simulink model "FocESMOGenerator"  (R2024a)
settings: Solver=FixedStepDiscrete  StartTime=0.0  StopTime=5  FixedStep=0.00005  RelTol=1e-3
values from neighbouring files (symbols this model uses):
  Ld = 5.135e-05    [ASMO_HFI_Generator.mat]
  Max_Current = 10    [ASMO_HFI_Generator.mat]
  Pole = 10    [ASMO_HFI_Generator.mat]
  Rs = 0.082    [ASMO_HFI_Generator.mat]
  Switch_Speed = 500    [ASMO_HFI_Generator.mat]
  UdInjectVal = 2.5    [ASMO_HFI_Generator.mat]
undefined symbols (not defined in the file or in its folder): DiscIntNeverNeededParam
libraries: slpidlib x5
(part 1 of 2)
settings Model: Creator=张先生  LastModifiedBy=张先生
settings OptimizationCC: DefaultParameterBehavior=Inlined  UseDivisionForNetSlopeComputation=on  GainParamInheritBuiltInType=on  UseFloatMulNetSlope=on  InlineInvariantSignals=on  PassReuseOutputArgsAs=Individual arguments  ZeroExternalMemoryAtStartup=off  ZeroInternalMemoryAtStartup=off  NoFixptDivByZeroProtection=on  EfficientFloat2IntCast=on  LifeSpan=1  OptimizeBlockOrder=speed  DifferentSizesBufferReuse=on  EfficientTunableParamExpr=on
settings DebuggingCC: ParameterTunabilityLossMsg=error
settings HardwareCC: ProdBitPerPointer=32  ProdBitPerSizeT=32  ProdBitPerPtrDiffT=32  ProdLargestAtomicInteger=Long  ProdLargestAtomicFloat=Double  ProdWordSize=32  ProdLongLongMode=on  ProdHWDeviceType=ARM Compatible->ARM Cortex-M
settings SFSimCC: MATLABDynamicMemAlloc=off
settings RTWCC: Description=Embedded Coder  SystemTargetFile=ert.tlc  GenCodeOnly=on  TemplateMakefile=ert_default_tmf  GenerateReport=on  LaunchReport=on
settings CodeAppCC: ForceParamTrailComments=on  IgnoreCustomStorageClasses=off  OperatorAnnotations=on  SimulinkDataObjDesc=on  SFDataObjDesc=on  CustomSymbolStrGlobalVar=rt$N$M  CustomSymbolStrType=$N$M  CustomSymbolStrFcn=$N$M$F  CustomSymbolStrMacro=$N$M  InsertBlockDesc=on
settings ERTTargetCC: TargetLangStandard=C99 (ISO)  CodeReplacementLibrary=ARM Cortex-M  GenerateSampleERTMain=on  IncludeMdlTerminateFcn=off  CombineSignalStateStructs=on  SupportComplex=off  SupportContinuousTime=on  InlinedParameterPlacement=NonHierarchical  ERTCustomFileTemplate=example_file_process.tlc  ERTFilePackagingFormat=CompactWithDataFile

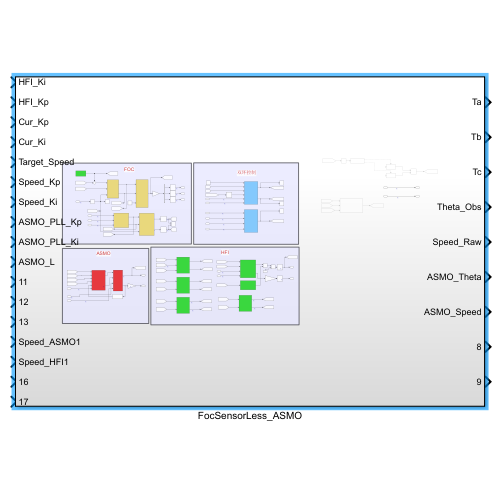
[thumbnail: Simulink's stored preview of the top-level diagram]
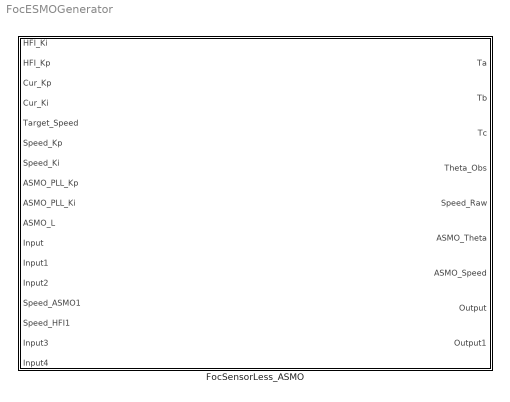
== system FocESMOGenerator ==
  FocSensorLess_ASMO : Subsystem

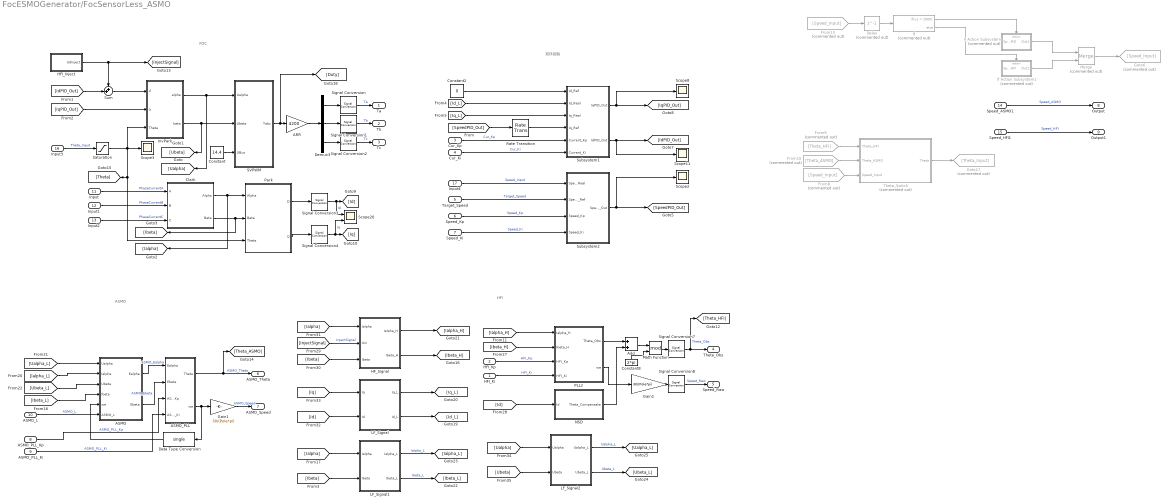
== system FocESMOGenerator/FocSensorLess_ASMO ==
  note: ASMO
  note: HFI
  note: 双环控制
  note: FOC
  HFI_Ki : Inport
  HFI_Kp : Inport  Port=2
  Cur_Kp : Inport  Port=3
  Cur_Ki : Inport  Port=4
  Target_Speed : Inport  Port=5
  Speed_Kp : Inport  Port=6
  Speed_Ki : Inport  Port=7
  ASMO_PLL_Kp : Inport  Port=8
  ASMO_PLL_Ki : Inport  Port=9
  ASMO_L : Inport  Port=10
  Input : Inport  Port=11
  Input1 : Inport  Port=12
  Input2 : Inport  Port=13
  Speed_ASMO1 : Inport  Port=14
  Speed_HFI1 : Inport  Port=15
  Input3 : Inport  Port=16
  Input4 : Inport  Port=17
  ARR : Gain  Gain=4200
  ASMO : Subsystem
  ASMO_PLL : Subsystem
  Add : Sum  OutDataTypeStr=single  AccumDataTypeStr=single
  Clark : Subsystem  TreatAsAtomicUnit=on
      settings: RTWSystemCode=Inline  RTWFcnNameOpts=Use subsystem name
      mask Display:
      | port_label('input',1,'a','texmode','on');
      | port_label('input',2,'b','texmode','on');
      | port_label('input',3,'c','texmode','on');
      | 
      | port_label('output',1,'\alpha','texmode','on');
      | port_label('output',2,'\beta','texmode','on');
      | 
      | fprintf('Clark');
  Constant : Constant  Value=14.4  OutDataTypeStr=single
  Constant2 : Constant  Value=0  OutDataTypeStr=single
  Constant8 : Constant  Value=2*pi  OutDataTypeStr=single
  Data Type Conversion : DataTypeConversion  OutDataTypeStr=single  SaturateOnIntegerOverflow=off  RndMeth=Floor
  Delay : Delay  Commented=on  DelayLength=1
  Demux3 : Demux  Outputs=3
  From10 : From  Commented=on  GotoTag=Theta_ASMO
  From13 : From  Commented=on  GotoTag=Speed_Input
  From8 : From  Commented=on  GotoTag=Speed_Input
  From9 : From  Commented=on  GotoTag=Theta_HFI
  Gain1 : Gain  Gain=30/(Pole*pi)
  Gain2 : Gain  Gain=30/(Pole*pi)  OutDataTypeStr=single
  Goto17 : Goto  Commented=on  GotoTag=Theta_Input
  Goto6 : Goto  Commented=on  GotoTag=Speed_Input
  HFI_Inject : Subsystem
  HF_Signal : Subsystem
  If : If  Commented=on  IfExpression=u1 > 1000
  If Action Subsystem : Subsystem  Commented=on  TreatAsAtomicUnit=on
  If Action Subsystem1 : Subsystem  Commented=on  TreatAsAtomicUnit=on
  InvPark : Subsystem  TreatAsAtomicUnit=on
      settings: RTWFcnNameOpts=Use subsystem name
      mask Display:
      | port_label('input',1,'d','texmode','on');
      | port_label('input',2,'q','texmode','on');
      | port_label('input',3,'\theta','texmode','on');
      | 
      | port_label('output',1,'\alpha','texmode','on');
      | port_label('output',2,'\beta','texmode','on');
      | 
      | fprintf('Inverse\nPark')
  LF_Signal : Subsystem
  LF_Signal1 : Subsystem
  LF_Signal2 : Subsystem
  Math Function : Math  Operator=mod
  Merge : Merge  Commented=on
  NSD : Subsystem
  PLL2 : Subsystem
  Park : Subsystem  TreatAsAtomicUnit=on
      settings: RTWFcnNameOpts=Use subsystem name
      mask Display:
      | port_label('input',1,'\alpha','texmode','on');
      | port_label('input',2, '\beta','texmode','on');
      | port_label('input',3, '\theta','texmode','on');
      | 
      | port_label('output',1,'d','texmode','on');
      | port_label('output',2,'q','texmode','on');
      | fprintf('Park');
  Rate Transition : RateTransition
  SVPWM : Subsystem  TreatAsAtomicUnit=on
  Saturation : Saturate  UpperLimit=2*pi-0.001  LowerLimit=-2*pi + 0.001
  Scope{2..3,8,11} (4 alike) : Scope
  Scope20 : Scope  NumInputPorts=2
  Signal Conversion{,1..4,7..8} (7 alike) : SignalConversion  OverrideOpt=off
  Subsystem1 : Subsystem
  Subsystem2 : Subsystem
  Sum : Sum  Inputs=++|
  Theta_Switch : Subsystem  Commented=on
  Ta : Outport
  Tb : Outport  Port=2
  Tc : Outport  Port=3
  Theta_Obs : Outport  Port=4
  Speed_Raw : Outport  Port=5
  ASMO_Theta : Outport  Port=6
  ASMO_Speed : Outport  Port=7
  Output : Outport  Port=8
  Output1 : Outport  Port=9
  wires:
  InvPark/1(alpha) -> SVPWM/1(Ualpha), [Ualpha]
  InvPark/2(beta) -> SVPWM/2(Ubeta), [Ubeta]
  Saturation/1 -> [Theta], Park/3(Theta), Scope3/1, InvPark/3(Theta)
  SVPWM/1(Tabc) -> [Duty], ARR/1
  ARR/1 -> Demux3/1
  Park/1(D) -> Signal Conversion3/1
  Signal Conversion4/1 -> Scope20/2, [Iq]  "Iq"
  Signal Conversion2/1 -> Tc/1  "Tc"
  Signal Conversion3/1 -> Scope20/1, [Id]  "Id"
  Signal Conversion/1 -> Ta/1  "Ta"
  Demux3/2 -> Signal Conversion1/1
  Demux3/1 -> Signal Conversion/1
  Park/2(Q) -> Signal Conversion4/1
  Demux3/3 -> Signal Conversion2/1
  Signal Conversion1/1 -> Tb/1  "Tb"
  Constant/1 -> SVPWM/3(UBus)
  Clark/2(Beta) -> [Ibeta], Park/2(Beta)
  Clark/1(Alpha) -> [Ialpha], Park/1(Alpha)
  [IqPID_Out] -> InvPark/2(q)
  Input3/1 -> Saturation/1  "Theta_Input"
  Gain1/1 -> ASMO_Speed/1  "ASMO_Speed"
  [Ialpha_L] -> ASMO/2(Ialpha)
  ASMO/2(Ebeta) -> ASMO_PLL/2(Ebeta)  "ASMO_Ebeta"
  ASMO_PLL/2(we) -> Gain1/1, Data Type Conversion/1
  ASMO/1(Ealpha) -> ASMO_PLL/1(Ealpha)  "ASMO_Ealpha"
  ASMO_PLL/1(Theta) -> [Theta_ASMO], ASMO_Theta/1  "ASMO_Theta"
  [Ualpha_L] -> ASMO/1(Ualpha)
  [Ubeta_L] -> ASMO/3(Ubeta)
  [Ibeta_L] -> ASMO/4(Ibeta)
  Data Type Conversion/1 -> ASMO/5(we)
  HFI_Inject/1(UdInject) -> Sum/1, [InjectSignal]
  [IdPID_Out] -> Sum/2
  Sum/1 -> InvPark/1(d)
  Gain2/1 -> Signal Conversion8/1
  [Ibeta_H] -> PLL2/2(Ibeta_H)
  PLL2/2(we) -> Gain2/1
  LF_Signal/2(Id_L) -> [Id_L]
  Add/1 -> Math Function/1
  [Id] -> NSD/1(Id)
  [Ialpha] -> HF_Signal/1(Ialpha)
  Signal Conversion8/1 -> Speed_Raw/1  "Speed_Raw"
  LF_Signal/1(Iq_L) -> [Iq_L]
  NSD/1(Theta_Compensate) -> Add/2
  HF_Signal/2(Ibeta_H) -> [Ibeta_H]
  [Ibeta] -> HF_Signal/3(Ibeta)
  [Id] -> LF_Signal/2(Id)
  HF_Signal/1(Ialpha_H) -> [Ialpha_H]
  [Iq] -> LF_Signal/1(Iq)
  HFI_Kp/1 -> PLL2/3(HFI_Kp)  "HFI_Kp"
  PLL2/1(Theta_Obs) -> Add/1
  Constant8/1 -> Math Function/2
  [Ialpha_H] -> PLL2/1(Ialpha_H)
  [InjectSignal] -> HF_Signal/2(Uin)  "InjectSignal"
  HFI_Ki/1 -> PLL2/4(HFI_Ki)  "HFI_Ki"
  Math Function/1 -> Signal Conversion7/1
  Signal Conversion7/1 -> [Theta_HFI], Theta_Obs/1  "Theta_Obs"
  [Iq_L] -> Subsystem1/3(Iq_Real)
  Cur_Kp/1 -> Subsystem1/5(Current_Kp)  "Cur_Kp"
  Speed_Kp/1 -> Subsystem2/3(Speed_Kp)  "Speed_Kp"
  Constant2/1 -> Subsystem1/1(Id_Ref)
  Subsystem2/1(SpeedPID_Out) -> Scope2/1, [SpeedPID_Out]
  Speed_Ki/1 -> Subsystem2/4(Speed_Ki)  "Speed_Ki"
  Input4/1 -> Subsystem2/1(Speed_Real)  "Speed_Input"
  [SpeedPID_Out] -> Rate Transition/1
  Cur_Ki/1 -> Subsystem1/6(Current_Ki)  "Cur_Ki"
  Rate Transition/1 -> Subsystem1/4(Iq_Ref)
  Target_Speed/1 -> Subsystem2/2(Speed_Ref)  "Target_Speed"
  Subsystem1/2(IdPID_Out) -> Scope11/1, [IdPID_Out]
  Subsystem1/1(IqPID_Out) -> Scope8/1, [IqPID_Out]
  [Id_L] -> Subsystem1/2(Id_Real)
  ASMO_PLL_Kp/1 -> ASMO_PLL/3(ASMO_PLL_Kp)  "ASMO_PLL_Kp"
  ASMO_PLL_Ki/1 -> ASMO_PLL/4(ASMO_PLL_Ki)  "ASMO_PLL_Ki"
  ASMO_L/1 -> ASMO/6(ASMO_L)  "ASMO_L"
  [Ibeta] -> LF_Signal1/2(Ibeta)
  [Ialpha] -> LF_Signal1/1(Ialpha)
  LF_Signal1/1(Ialpha_L) -> [Ialpha_L]  "Ialpha_L"
  LF_Signal1/2(Ibeta_L) -> [Ibeta_L]  "Ibeta_L"
  [Ubeta] -> LF_Signal2/2(Ubeta)
  LF_Signal2/2(Ubeta_L) -> [Ubeta_L]  "Ubeta_L"
  LF_Signal2/1(Ualpha_L) -> [Ualpha_L]  "Ualpha_L"
  [Ualpha] -> LF_Signal2/1(Ualpha)
  Input/1 -> Clark/1(A)  "PhaseCurrentA"
  Input2/1 -> Clark/3(C)  "PhaseCurrentC"
  Input1/1 -> Clark/2(B)  "PhaseCurrentB"
  From8/1 -> Theta_Switch/3(Speed_Input)
  From10/1 -> Theta_Switch/2(Theta_ASMO)
  From9/1 -> Theta_Switch/1(Theta_HFI)
  Theta_Switch/1(Theta) -> Goto17/1
  If/1 -> If Action Subsystem/Action
  If/2 -> If Action Subsystem1/Action
  If Action Subsystem/1(Out1) -> Merge/1
  If Action Subsystem1/1(Out1) -> Merge/2
  Merge/1 -> Goto6/1
  From13/1 -> Delay/1
  Delay/1 -> If/1
  Speed_HFI1/1 -> Output1/1  "Speed_HFI"
  Speed_ASMO1/1 -> Output/1  "Speed_ASMO"

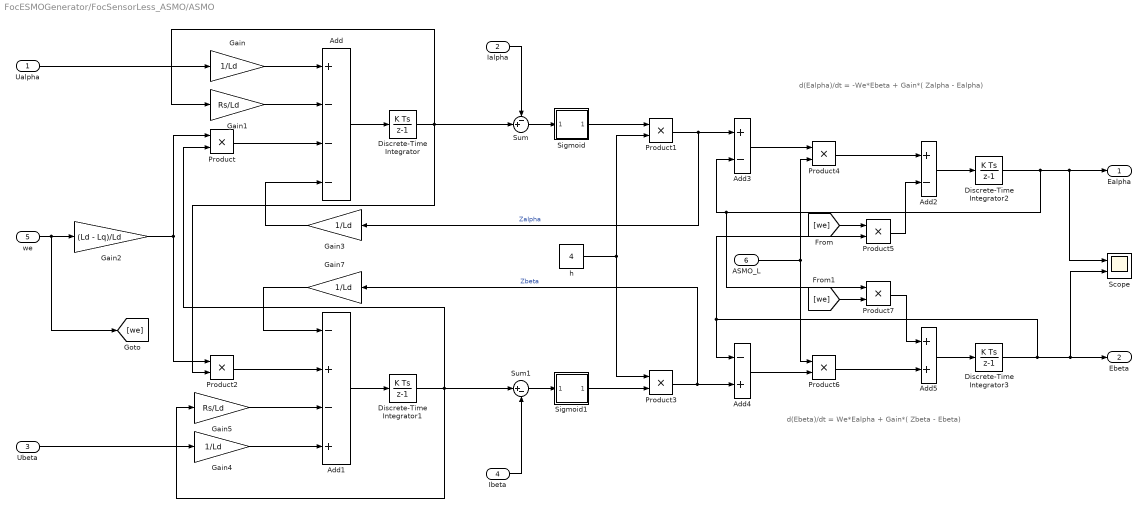
== system FocESMOGenerator/FocSensorLess_ASMO/ASMO ==
  note: d(Ealpha)/dt = -We*Ebeta + Gain*( Zalpha - Ealpha)
  note: d(Ebeta)/dt = We*Ealpha + Gain*( Zbeta - Ebeta)
  Ualpha : Inport
  Ialpha : Inport  Port=2
  Ubeta : Inport  Port=3
  Ibeta : Inport  Port=4
  we : Inport  Port=5
  ASMO_L : Inport  Port=6
  Add : Sum  Inputs=+---  OutDataTypeStr=single  AccumDataTypeStr=single
  Add1 : Sum  Inputs=-+-+  OutDataTypeStr=single  AccumDataTypeStr=single
  Add2 : Sum  Inputs=+-  OutDataTypeStr=single  AccumDataTypeStr=single
  Add3 : Sum  Inputs=+-  OutDataTypeStr=single  AccumDataTypeStr=single
  Add4 : Sum  Inputs=-+  OutDataTypeStr=single  AccumDataTypeStr=single
  Add5 : Sum  OutDataTypeStr=single  AccumDataTypeStr=single
  Discrete-Time Integrator{,1..3} (4 alike) : DiscreteIntegrator  SampleTime=-1  OutDataTypeStr=single  ICPrevOutput=DiscIntNeverNeededParam  ICPrevScaledInput=DiscIntNeverNeededParam
  Gain{,3..4,7} (4 alike) : Gain  Gain=1/Ld  OutDataTypeStr=single
  Gain1 : Gain  Gain=Rs/Ld  OutDataTypeStr=single
  Gain2 : Gain  Gain=(Ld - Lq)/Ld
  Gain5 : Gain  Gain=Rs/Ld  OutDataTypeStr=single
  Product{,1..6} (7 alike) : Product  OutDataTypeStr=single
  Product7 : Product
  Scope : Scope  NumInputPorts=2
  Sigmoid : Subsystem
  Sigmoid1 : Subsystem
  Sum : Sum  Inputs=-+|
  Sum1 : Sum  Inputs=|+-
  h : Constant  Value=4  OutDataTypeStr=single
  Ealpha : Outport
  Ebeta : Outport  Port=2
  wires:
  Gain/1 -> Add/1
  Gain1/1 -> Add/2
  Ualpha/1 -> Gain/1
  Add/1 -> Discrete-Time Integrator/1
  Product/1 -> Add/3
  Gain2/1 -> Product2/1, Product/1
  Discrete-Time Integrator/1 -> Product2/2, Sum/2, Gain1/1
  Ialpha/1 -> Sum/1
  Sum/1 -> Sigmoid/1(In1)
  Sigmoid/1(Out1) -> Product1/1
  h/1 -> Product3/1, Product1/2
  Product1/1 -> Add3/1, Gain3/1  "Zalpha"
  Gain3/1 -> Add/4
  Add1/1 -> Discrete-Time Integrator1/1
  Product3/1 -> Add4/2, Gain7/1  "Zbeta"
  Sum1/1 -> Sigmoid1/1(In1)
  Discrete-Time Integrator1/1 -> Sum1/1, Gain5/1, Product/2
  Ibeta/1 -> Sum1/2
  Sigmoid1/1(Out1) -> Product3/2
  Gain4/1 -> Add1/4
  Gain5/1 -> Add1/3
  Product2/1 -> Add1/2
  Gain7/1 -> Add1/1
  Ubeta/1 -> Gain4/1
  Add3/1 -> Product4/1
  Product4/1 -> Add2/1
  Add2/1 -> Discrete-Time Integrator2/1
  Discrete-Time Integrator2/1 -> Ealpha/1, Scope/1, Product7/1, Add3/2
  ASMO_L/1 -> Product4/2, Product6/1
  Product5/1 -> Add2/2
  [we] -> Product5/1
  Add4/1 -> Product6/2
  Product6/1 -> Add5/2
  [we] -> Product7/2
  Product7/1 -> Add5/1
  Add5/1 -> Discrete-Time Integrator3/1
  Discrete-Time Integrator3/1 -> Product5/2, Add4/1, Scope/2, Ebeta/1
  we/1 -> [we], Gain2/1

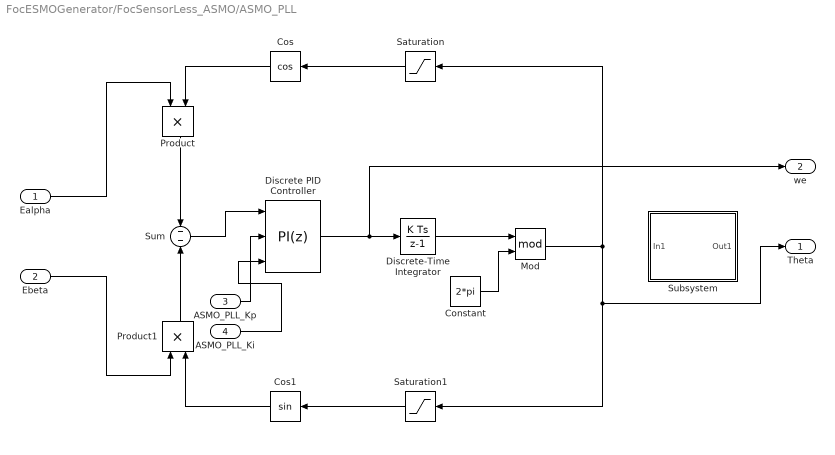
== system FocESMOGenerator/FocSensorLess_ASMO/ASMO_PLL ==
  Ealpha : Inport
  Ebeta : Inport  Port=2
  ASMO_PLL_Kp : Inport  Port=3
  ASMO_PLL_Ki : Inport  Port=4
  Constant : Constant  Value=2*pi  OutDataTypeStr=single
  Cos : Trigonometry  Operator=cos  ApproximationMethod=Lookup
  Cos1 : Trigonometry  ApproximationMethod=Lookup
  Discrete PID Controller : slpidlib/PID Controller  Controller=PI  Form=Parallel  TimeDomain=Discrete-time  UseExternalTs=off  SampleTime=-1  IntegratorMethod=Forward Euler  FilterMethod=Forward Euler  ControllerParametersSource=external  P=10  I=1000  UseKiTs=off  D=0  UseExternalDerivativeSource=off  N=100  UseFilter=on  TunerSelectOption=Transfer Function Based (PID Tuner App)  InitialConditionSource=internal  InitialConditionForIntegrator=0  InitialConditionForFilter=0  DifferentiatorICPrevScaledInput=0  ExternalReset=none  TrackingMode=off  Kt=1  LimitOutput=off  SatLimitsSource=internal  UpperSaturationLimit=pi*2  LowerSaturationLimit=-pi*2  LinearizeAsGain=on  AntiWindupMode=clamping  Kb=1  LimitIntegrator=off  UpperIntegratorSaturationLimit=inf  LowerIntegratorSaturationLimit=-inf  PGainOutDataTypeStr=single  PProdOutDataTypeStr=single  POutMin=[]  POutMax=[]  IGainOutDataTypeStr=single  IProdOutDataTypeStr=single  IOutMin=[]  IOutMax=[]  DOutMin=[]  DOutMax=[]  NOutMin=[]  NOutMax=[]  SumOutDataTypeStr=single  SumOutMin=[]  SumOutMax=[]  SaturationOutMin=[]  SaturationOutMax=[]  PParamMin=[]  PParamMax=[]  IParamMin=[]  IParamMax=[]  DParamMin=[]  DParamMax=[]  NParamMin=[]  NParamMax=[]  KbParamMin=[]  KbParamMax=[]  KtParamMin=[]  KtParamMax=[]  KbOutMin=[]  KbOutMax=[]  KtOutMin=[]  KtOutMax=[]  IntegratorOutMin=[]  IntegratorOutMax=[]  FilterOutMin=[]  FilterOutMax=[]  SumI1OutMin=[]  SumI1OutMax=[]  SumI2OutMin=[]  SumI2OutMax=[]  SumI3OutMin=[]  SumI3OutMax=[]  SumI4OutMin=[]  SumI4OutMax=[]  SumDOutMin=[]  SumDOutMax=[]  DifferentiatorOutMin=[]  DifferentiatorOutMax=[]  FilterDiffOutCoefMin=[]  FilterDiffOutCoefMax=[]  ReciprocalOutMin=[]  ReciprocalOutMax=[]  SumDenOutMin=[]  SumDenOutMax=[]  SumNumOutMin=[]  SumNumOutMax=[]  DivideOutMin=[]  DivideOutMax=[]  UdiffTsProdOutMin=[]  UdiffTsProdOutMax=[]  NTsProdOutMin=[]  NTsProdOutMax=[]  UintegralTsProdOutMin=[]  UintegralTsProdOutMax=[]  UngainTsProdOutMin=[]  UngainTsProdOutMax=[]  ClampingZeroOutDataTypeStr=Inherit: Inherit via back propagation  ClampingZeroOutMin=[]  ClampingZeroOutMax=[]  FilterDenConstantOutDataTypeStr=Inherit: Inherit via back propagation  FilterDenConstantOutMin=[]  FilterDenConstantOutMax=[]  PCopyOutDataTypeStr=Inherit: Inherit via back propagation  PCopyOutMin=[]  PCopyOutMax=[]  NCopyOutDataTypeStr=Inherit: Inherit via back propagation  NCopyOutMin=[]  NCopyOutMax=[]  IntegratorContinuousStateAttributes=''  IntegratorStateMustResolveToSignalObject=off  IntegratorRTWStateStorageClass=Auto  FilterContinuousStateAttributes=''  FilterStateMustResolveToSignalObject=off  FilterRTWStateStorageClass=Auto  ParallelPVariant=ExternalParameters  IdealPVariant=Disabled  IVariant=ExternalParameters  DVariant=Disabled  IntegratorVariant=Discrete  SatVariant=Disabled  AWVariant=Passthrough  PCopyVariant=Disabled  TRVariant=Disabled  FdbkBlocksVariant=Forward  IdealPFdbkVariant=Disabled  SatFdbkVariant=Disabled  DerivativeFilterVariant=Disabled  NVariant=Disabled  NCopyVariant=Disabled_SignalSpec  FilterICVariant=Disabled  IntegratorICVariant=InternalICs  ExternalResetVariant=Disabled  TRSumVariant=Passthrough  SumFdbkVariant=Disabled  SumVariant=Sum_PI  TsampFilterVariant=InternalTs  TsampNgainVariant=Passthrough  TsampIntegralVariant=Disabled_SignalSpec  ExternalSaturationOutDataTypeStr=Inherit: Same as second input  DerivativeSourceVariant=Disabled
      settings: LibrarySourceBlock=simulink/Discrete/Discrete PID Controller
  Discrete-Time Integrator : DiscreteIntegrator  SampleTime=-1  OutDataTypeStr=single  ICPrevOutput=DiscIntNeverNeededParam  ICPrevScaledInput=DiscIntNeverNeededParam
  Mod : Math  Operator=mod
  Product : Product  OutDataTypeStr=single
  Product1 : Product  OutDataTypeStr=single
  Saturation : Saturate  UpperLimit=2*pi - 0.001  LowerLimit=-2*pi + 0.001
  Saturation1 : Saturate  UpperLimit=2*pi - 0.001  LowerLimit=-2*pi + 0.001
  Subsystem : Subsystem
  Sum : Sum  Inputs=-|-
  Theta : Outport
  we : Outport  Port=2
  wires:
  Ebeta/1 -> Product1/1
  Ealpha/1 -> Product/1
  Product/1 -> Sum/1
  Product1/1 -> Sum/2
  Sum/1 -> Discrete PID Controller/1
  Discrete-Time Integrator/1 -> Mod/1
  Constant/1 -> Mod/2
  Mod/1 -> Theta/1, Saturation1/1, Saturation/1
  Saturation/1 -> Cos/1
  Cos/1 -> Product/2
  Saturation1/1 -> Cos1/1
  Cos1/1 -> Product1/2
  Discrete PID Controller/1 -> we/1, Discrete-Time Integrator/1
  ASMO_PLL_Kp/1 -> Discrete PID Controller/2
  ASMO_PLL_Ki/1 -> Discrete PID Controller/3

== system FocESMOGenerator/FocSensorLess_ASMO/Clark ==
  A : Inport  OutDataTypeStr=single
  B : Inport  Port=2  OutDataTypeStr=single
  C : Inport  Port=3  OutDataTypeStr=single
  Gain : Gain  Gain=single(2/3)  OutDataTypeStr=single
  Gain1 : Gain  Gain=0.5  OutDataTypeStr=single
  Gain2 : Gain  Gain=single(sqrt(3)/3)  OutDataTypeStr=single
  Sum : Sum  Inputs=|++  OutDataTypeStr=single
  Sum1 : Sum  Inputs=|+-  OutDataTypeStr=single
  Sum2 : Sum  Inputs=+-|  OutDataTypeStr=single
  Alpha : Outport  OutDataTypeStr=single
  Beta : Outport  Port=2  OutDataTypeStr=single
  wires:
  Sum/1 -> Gain1/1
  Gain2/1 -> Beta/1
  B/1 -> Sum2/1, Sum/1
  Gain1/1 -> Sum1/2
  Gain/1 -> Alpha/1
  Sum2/1 -> Gain2/1
  C/1 -> Sum2/2, Sum/2
  A/1 -> Sum1/1
  Sum1/1 -> Gain/1

== system FocESMOGenerator/FocSensorLess_ASMO/HFI_Inject ==
  note: 前0.2S进行极性辨识
  Scope : Scope
  Scope1 : Scope  NumInputPorts=2
  Subsystem : Subsystem
  Subsystem4 : Subsystem
  Sum1 : Sum  Inputs=++|
  UdInject : Outport
  wires:
  Subsystem/1(Ud_Inject) -> Scope1/2, Sum1/2
  Subsystem4/1(NDS_Signal) -> Scope1/1, Sum1/1
  Sum1/1 -> Scope/1, UdInject/1

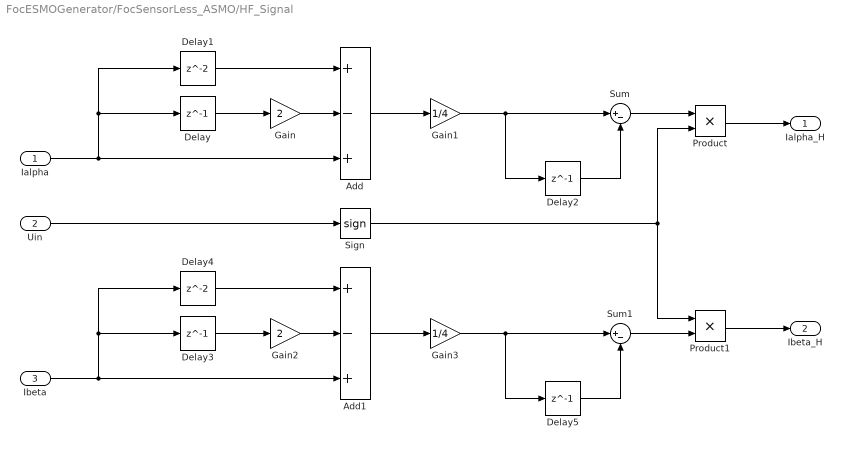
== system FocESMOGenerator/FocSensorLess_ASMO/HF_Signal ==
  Ialpha : Inport
  Uin : Inport  Port=2
  Ibeta : Inport  Port=3
  Add : Sum  Inputs=+-+  OutDataTypeStr=single  AccumDataTypeStr=single
  Add1 : Sum  Inputs=+-+  OutDataTypeStr=single  AccumDataTypeStr=single
  Delay{,2..3,5} (4 alike) : Delay  DelayLength=1
  Delay1 : Delay
  Delay4 : Delay
  Gain : Gain  Gain=2  OutDataTypeStr=single
  Gain1 : Gain  Gain=1/4  OutDataTypeStr=single
  Gain2 : Gain  Gain=2  OutDataTypeStr=single
  Gain3 : Gain  Gain=1/4  OutDataTypeStr=single
  Product : Product  OutDataTypeStr=single
  Product1 : Product  OutDataTypeStr=single
  Sign : Signum
  Sum : Sum  Inputs=|+-
  Sum1 : Sum  Inputs=|+-
  Ialpha_H : Outport
  Ibeta_H : Outport  Port=2
  wires:
  Delay/1 -> Gain/1
  Delay1/1 -> Add/1
  Gain/1 -> Add/2
  Ialpha/1 -> Add/3, Delay1/1, Delay/1
  Add/1 -> Gain1/1
  Gain1/1 -> Delay2/1, Sum/1
  Delay2/1 -> Sum/2
  Sum/1 -> Product/1
  Product/1 -> Ialpha_H/1
  Uin/1 -> Sign/1
  Sign/1 -> Product1/1, Product/2
  Product1/1 -> Ibeta_H/1
  Add1/1 -> Gain3/1
  Delay5/1 -> Sum1/2
  Gain3/1 -> Delay5/1, Sum1/1
  Delay4/1 -> Add1/1
  Gain2/1 -> Add1/2
  Ibeta/1 -> Add1/3, Delay4/1, Delay3/1
  Delay3/1 -> Gain2/1
  Sum1/1 -> Product1/2

== system FocESMOGenerator/FocSensorLess_ASMO/If Action Subsystem ==
  Speed_ASMO : Inport
  Action Port : ActionPort  ActionPortLabel=if(u1 > 1000)
  Out1 : Outport
  wires:
  Speed_ASMO/1 -> Out1/1

== system FocESMOGenerator/FocSensorLess_ASMO/If Action Subsystem1 ==
  Speed_HFI : Inport
  Action Port : ActionPort  ActionPortLabel=else
  Out1 : Outport
  wires:
  Speed_HFI/1 -> Out1/1

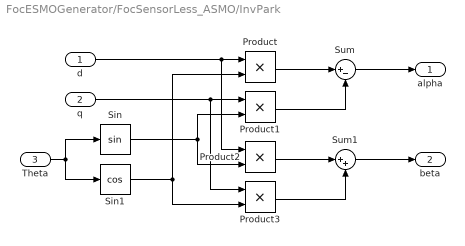
== system FocESMOGenerator/FocSensorLess_ASMO/InvPark ==
  d : Inport  OutDataTypeStr=single
  q : Inport  Port=2  OutDataTypeStr=single
  Theta : Inport  Port=3  OutDataTypeStr=single
  Product{,1..3} (4 alike) : Product  OutDataTypeStr=single
  Sin : Trigonometry  ApproximationMethod=Lookup  TableDataTypeStr=single
  Sin1 : Trigonometry  Operator=cos  ApproximationMethod=Lookup  TableDataTypeStr=single
  Sum : Sum  Inputs=|+-  OutDataTypeStr=single
  Sum1 : Sum  Inputs=|++  OutDataTypeStr=single
  alpha : Outport  OutDataTypeStr=single
  beta : Outport  Port=2  OutDataTypeStr=single
  wires:
  Sum/1 -> alpha/1
  Theta/1 -> Sin1/1, Sin/1
  d/1 -> Product2/1, Product/1
  Sin1/1 -> Product/2, Product3/2
  q/1 -> Product3/1, Product1/1
  Sin/1 -> Product1/2, Product2/2
  Product/1 -> Sum/1
  Product1/1 -> Sum/2
  Product2/1 -> Sum1/1
  Product3/1 -> Sum1/2
  Sum1/1 -> beta/1

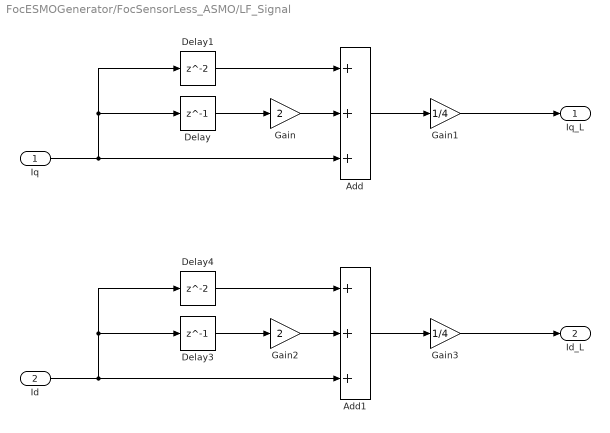
== system FocESMOGenerator/FocSensorLess_ASMO/LF_Signal ==
  Iq : Inport
  Id : Inport  Port=2
  Add : Sum  Inputs=+++  OutDataTypeStr=single  AccumDataTypeStr=single
  Add1 : Sum  Inputs=+++  OutDataTypeStr=single  AccumDataTypeStr=single
  Delay : Delay  DelayLength=1
  Delay1 : Delay
  Delay3 : Delay  DelayLength=1
  Delay4 : Delay
  Gain : Gain  Gain=2
  Gain1 : Gain  Gain=1/4  OutDataTypeStr=single
  Gain2 : Gain  Gain=2
  Gain3 : Gain  Gain=1/4  OutDataTypeStr=single
  Iq_L : Outport
  Id_L : Outport  Port=2
  wires:
  Delay/1 -> Gain/1
  Delay1/1 -> Add/1
  Gain/1 -> Add/2
  Iq/1 -> Add/3, Delay1/1, Delay/1
  Add/1 -> Gain1/1
  Gain1/1 -> Iq_L/1
  Gain3/1 -> Id_L/1
  Add1/1 -> Gain3/1
  Delay4/1 -> Add1/1
  Gain2/1 -> Add1/2
  Id/1 -> Add1/3, Delay4/1, Delay3/1
  Delay3/1 -> Gain2/1

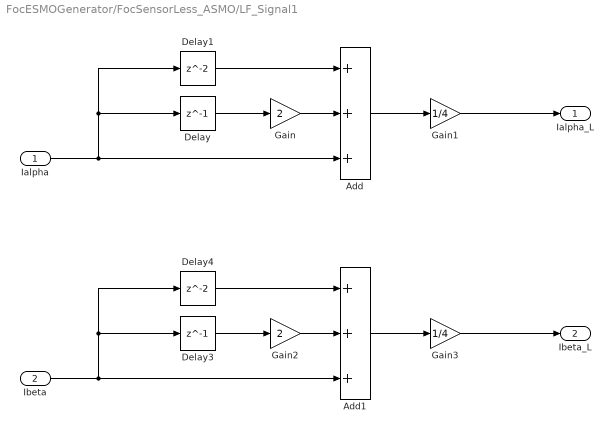
== system FocESMOGenerator/FocSensorLess_ASMO/LF_Signal1 ==
  Ialpha : Inport
  Ibeta : Inport  Port=2
  Add : Sum  Inputs=+++  OutDataTypeStr=single  AccumDataTypeStr=single
  Add1 : Sum  Inputs=+++  OutDataTypeStr=single  AccumDataTypeStr=single
  Delay : Delay  DelayLength=1
  Delay1 : Delay
  Delay3 : Delay  DelayLength=1
  Delay4 : Delay
  Gain : Gain  Gain=2  OutDataTypeStr=single
  Gain1 : Gain  Gain=1/4  OutDataTypeStr=single
  Gain2 : Gain  Gain=2  OutDataTypeStr=single
  Gain3 : Gain  Gain=1/4  OutDataTypeStr=single
  Ialpha_L : Outport
  Ibeta_L : Outport  Port=2
  wires:
  Delay/1 -> Gain/1
  Delay1/1 -> Add/1
  Gain/1 -> Add/2
  Ialpha/1 -> Add/3, Delay1/1, Delay/1
  Add/1 -> Gain1/1
  Gain1/1 -> Ialpha_L/1
  Gain3/1 -> Ibeta_L/1
  Add1/1 -> Gain3/1
  Delay4/1 -> Add1/1
  Gain2/1 -> Add1/2
  Ibeta/1 -> Add1/3, Delay4/1, Delay3/1
  Delay3/1 -> Gain2/1

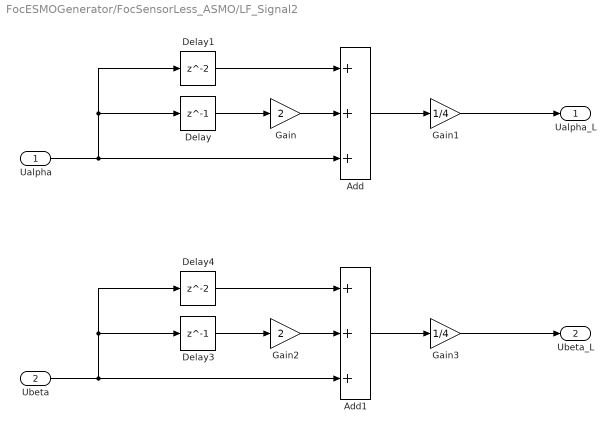
== system FocESMOGenerator/FocSensorLess_ASMO/LF_Signal2 ==
  Ualpha : Inport
  Ubeta : Inport  Port=2
  Add : Sum  Inputs=+++  OutDataTypeStr=single  AccumDataTypeStr=single
  Add1 : Sum  Inputs=+++  OutDataTypeStr=single  AccumDataTypeStr=single
  Delay : Delay  DelayLength=1
  Delay1 : Delay
  Delay3 : Delay  DelayLength=1
  Delay4 : Delay
  Gain : Gain  Gain=2  OutDataTypeStr=single
  Gain1 : Gain  Gain=1/4  OutDataTypeStr=single
  Gain2 : Gain  Gain=2  OutDataTypeStr=single
  Gain3 : Gain  Gain=1/4  OutDataTypeStr=single
  Ualpha_L : Outport
  Ubeta_L : Outport  Port=2
  wires:
  Delay/1 -> Gain/1
  Delay1/1 -> Add/1
  Gain/1 -> Add/2
  Ualpha/1 -> Add/3, Delay1/1, Delay/1
  Add/1 -> Gain1/1
  Gain1/1 -> Ualpha_L/1
  Gain3/1 -> Ubeta_L/1
  Add1/1 -> Gain3/1
  Delay4/1 -> Add1/1
  Gain2/1 -> Add1/2
  Ubeta/1 -> Add1/3, Delay4/1, Delay3/1
  Delay3/1 -> Gain2/1

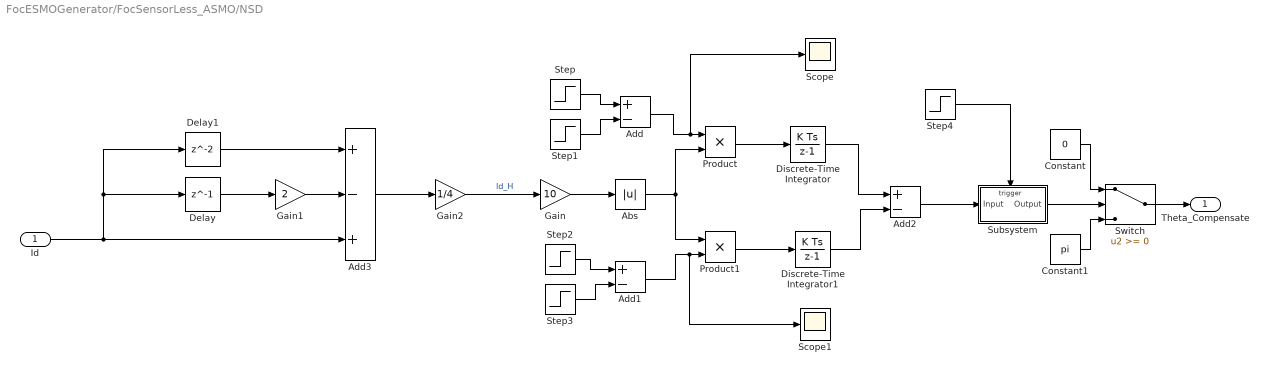
== system FocESMOGenerator/FocSensorLess_ASMO/NSD ==
  Id : Inport
  Abs : Abs  OutDataTypeStr=single  SaturateOnIntegerOverflow=off
  Add : Sum  Inputs=+-  OutDataTypeStr=single  AccumDataTypeStr=single
  Add1 : Sum  Inputs=+-  OutDataTypeStr=single  AccumDataTypeStr=single
  Add2 : Sum  Inputs=+-  OutDataTypeStr=single  AccumDataTypeStr=single
  Add3 : Sum  Inputs=+-+  OutDataTypeStr=single  AccumDataTypeStr=single
  Constant : Constant  Value=0  OutDataTypeStr=single
  Constant1 : Constant  Value=pi  OutDataTypeStr=single
  Delay : Delay  DelayLength=1
  Delay1 : Delay
  Discrete-Time Integrator : DiscreteIntegrator  SampleTime=-1  OutDataTypeStr=single  ICPrevOutput=DiscIntNeverNeededParam  ICPrevScaledInput=DiscIntNeverNeededParam
  Discrete-Time Integrator1 : DiscreteIntegrator  SampleTime=-1  OutDataTypeStr=single  ICPrevOutput=DiscIntNeverNeededParam  ICPrevScaledInput=DiscIntNeverNeededParam
  Gain : Gain  Gain=10  OutDataTypeStr=single
  Gain1 : Gain  Gain=2  OutDataTypeStr=single
  Gain2 : Gain  Gain=1/4  OutDataTypeStr=single
  Product : Product  OutDataTypeStr=single
  Product1 : Product  OutDataTypeStr=single
  Scope : Scope
  Scope1 : Scope
  Step : Step  Time=0.1  OutDataTypeStr=single  SampleTime=0
  Step1 : Step  Time=0.11  OutDataTypeStr=single  SampleTime=0
  Step2 : Step  Time=0.13  After=-1  OutDataTypeStr=single  SampleTime=0
  Step3 : Step  Time=0.14  After=-1  OutDataTypeStr=single  SampleTime=0
  Step4 : Step  Time=0.15  OutDataTypeStr=single  SampleTime=0
  Subsystem : Subsystem
  Switch : Switch  OutDataTypeStr=single  SaturateOnIntegerOverflow=off  InputSameDT=off
  Theta_Compensate : Outport
  wires:
  Gain/1 -> Abs/1
  Step/1 -> Add/1
  Step1/1 -> Add/2
  Step2/1 -> Add1/1
  Step3/1 -> Add1/2
  Add/1 -> Scope/1, Product/1
  Add1/1 -> Scope1/1, Product1/2
  Abs/1 -> Product1/1, Product/2
  Product/1 -> Discrete-Time Integrator/1
  Product1/1 -> Discrete-Time Integrator1/1
  Discrete-Time Integrator/1 -> Add2/1
  Discrete-Time Integrator1/1 -> Add2/2
  Step4/1 -> Subsystem/Trigger
  Add2/1 -> Subsystem/1(Input)
  Subsystem/1(Output) -> Switch/2
  Constant/1 -> Switch/1
  Constant1/1 -> Switch/3
  Switch/1 -> Theta_Compensate/1
  Id/1 -> Add3/3, Delay1/1, Delay/1
  Gain1/1 -> Add3/2
  Delay1/1 -> Add3/1
  Add3/1 -> Gain2/1
  Delay/1 -> Gain1/1
  Gain2/1 -> Gain/1  "Id_H"

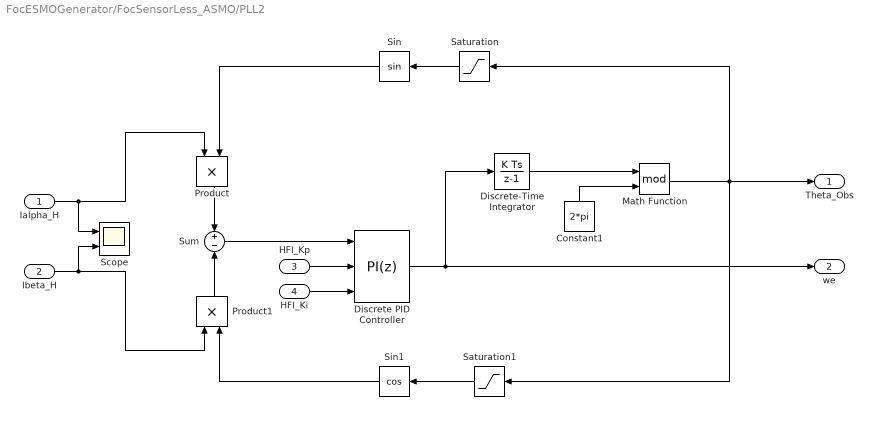
== system FocESMOGenerator/FocSensorLess_ASMO/PLL2 ==
  Ialpha_H : Inport
  Ibeta_H : Inport  Port=2
  HFI_Kp : Inport  Port=3
  HFI_Ki : Inport  Port=4
  Constant1 : Constant  Value=2*pi  OutDataTypeStr=single
  Discrete PID Controller : slpidlib/PID Controller  Controller=PI  Form=Parallel  TimeDomain=Discrete-time  UseExternalTs=off  SampleTime=-1  IntegratorMethod=Forward Euler  FilterMethod=Forward Euler  ControllerParametersSource=external  P=10  I=1000  UseKiTs=off  D=0  UseExternalDerivativeSource=off  N=100  UseFilter=on  TunerSelectOption=Transfer Function Based (PID Tuner App)  InitialConditionSource=internal  InitialConditionForIntegrator=0  InitialConditionForFilter=0  DifferentiatorICPrevScaledInput=0  ExternalReset=none  TrackingMode=off  Kt=1  LimitOutput=off  SatLimitsSource=internal  UpperSaturationLimit=pi*2  LowerSaturationLimit=-pi*2  LinearizeAsGain=on  AntiWindupMode=clamping  Kb=1  LimitIntegrator=off  UpperIntegratorSaturationLimit=inf  LowerIntegratorSaturationLimit=-inf  PGainOutDataTypeStr=single  PProdOutDataTypeStr=single  POutMin=[]  POutMax=[]  IGainOutDataTypeStr=single  IProdOutDataTypeStr=single  IOutMin=[]  IOutMax=[]  DOutMin=[]  DOutMax=[]  NOutMin=[]  NOutMax=[]  SumOutDataTypeStr=single  SumOutMin=[]  SumOutMax=[]  SaturationOutMin=[]  SaturationOutMax=[]  PParamMin=[]  PParamMax=[]  IParamMin=[]  IParamMax=[]  DParamMin=[]  DParamMax=[]  NParamMin=[]  NParamMax=[]  KbParamMin=[]  KbParamMax=[]  KtParamMin=[]  KtParamMax=[]  KbOutMin=[]  KbOutMax=[]  KtOutMin=[]  KtOutMax=[]  IntegratorOutMin=[]  IntegratorOutMax=[]  FilterOutMin=[]  FilterOutMax=[]  SumI1OutMin=[]  SumI1OutMax=[]  SumI2OutMin=[]  SumI2OutMax=[]  SumI3OutMin=[]  SumI3OutMax=[]  SumI4OutMin=[]  SumI4OutMax=[]  SumDOutMin=[]  SumDOutMax=[]  DifferentiatorOutMin=[]  DifferentiatorOutMax=[]  FilterDiffOutCoefMin=[]  FilterDiffOutCoefMax=[]  ReciprocalOutMin=[]  ReciprocalOutMax=[]  SumDenOutMin=[]  SumDenOutMax=[]  SumNumOutMin=[]  SumNumOutMax=[]  DivideOutMin=[]  DivideOutMax=[]  UdiffTsProdOutMin=[]  UdiffTsProdOutMax=[]  NTsProdOutMin=[]  NTsProdOutMax=[]  UintegralTsProdOutMin=[]  UintegralTsProdOutMax=[]  UngainTsProdOutMin=[]  UngainTsProdOutMax=[]  ClampingZeroOutDataTypeStr=Inherit: Inherit via back propagation  ClampingZeroOutMin=[]  ClampingZeroOutMax=[]  FilterDenConstantOutDataTypeStr=Inherit: Inherit via back propagation  FilterDenConstantOutMin=[]  FilterDenConstantOutMax=[]  PCopyOutDataTypeStr=Inherit: Inherit via back propagation  PCopyOutMin=[]  PCopyOutMax=[]  NCopyOutDataTypeStr=Inherit: Inherit via back propagation  NCopyOutMin=[]  NCopyOutMax=[]  IntegratorContinuousStateAttributes=''  IntegratorStateMustResolveToSignalObject=off  IntegratorRTWStateStorageClass=Auto  FilterContinuousStateAttributes=''  FilterStateMustResolveToSignalObject=off  FilterRTWStateStorageClass=Auto  ParallelPVariant=ExternalParameters  IdealPVariant=Disabled  IVariant=ExternalParameters  DVariant=Disabled  IntegratorVariant=Discrete  SatVariant=Disabled  AWVariant=Passthrough  PCopyVariant=Disabled  TRVariant=Disabled  FdbkBlocksVariant=Forward  IdealPFdbkVariant=Disabled  SatFdbkVariant=Disabled  DerivativeFilterVariant=Disabled  NVariant=Disabled  NCopyVariant=Disabled_SignalSpec  FilterICVariant=Disabled  IntegratorICVariant=InternalICs  ExternalResetVariant=Disabled  TRSumVariant=Passthrough  SumFdbkVariant=Disabled  SumVariant=Sum_PI  TsampFilterVariant=InternalTs  TsampNgainVariant=Passthrough  TsampIntegralVariant=Disabled_SignalSpec  ExternalSaturationOutDataTypeStr=Inherit: Same as second input  DerivativeSourceVariant=Disabled
      settings: LibrarySourceBlock=simulink/Discrete/Discrete PID Controller
  Discrete-Time Integrator : DiscreteIntegrator  SampleTime=-1  OutDataTypeStr=single  ICPrevOutput=DiscIntNeverNeededParam  ICPrevScaledInput=DiscIntNeverNeededParam
  Math Function : Math  Operator=mod
  Product : Product
  Product1 : Product
  Saturation : Saturate  UpperLimit=2*pi - 0.001  LowerLimit=-2*pi + 0.001  OutDataTypeStr=single
  Saturation1 : Saturate  UpperLimit=2*pi - 0.001  LowerLimit=-2*pi + 0.001  OutDataTypeStr=single
  Scope : Scope  NumInputPorts=2
  Sin : Trigonometry  ApproximationMethod=Lookup
  Sin1 : Trigonometry  Operator=cos  ApproximationMethod=Lookup
  Sum : Sum  Inputs=+|-
  Theta_Obs : Outport
  we : Outport  Port=2
  wires:
  Product/1 -> Sum/1
  Product1/1 -> Sum/2
  Ialpha_H/1 -> Product/1, Scope/1
  Ibeta_H/1 -> Scope/2, Product1/1
  Sum/1 -> Discrete PID Controller/1
  Discrete PID Controller/1 -> Discrete-Time Integrator/1, we/1
  Discrete-Time Integrator/1 -> Math Function/1
  Sin/1 -> Product/2
  Sin1/1 -> Product1/2
  Saturation/1 -> Sin/1
  Saturation1/1 -> Sin1/1
  Constant1/1 -> Math Function/2
  Math Function/1 -> Theta_Obs/1, Saturation/1, Saturation1/1
  HFI_Kp/1 -> Discrete PID Controller/2
  HFI_Ki/1 -> Discrete PID Controller/3

== system FocESMOGenerator/FocSensorLess_ASMO/Park ==
  Alpha : Inport  OutDataTypeStr=single
  Beta : Inport  Port=2  OutDataTypeStr=single
  Theta : Inport  Port=3  OutDataTypeStr=single
  Product{,1..3} (4 alike) : Product  OutDataTypeStr=single
  Sin : Trigonometry  ApproximationMethod=Lookup  TableDataTypeStr=single
  Sin1 : Trigonometry  Operator=cos  ApproximationMethod=Lookup  TableDataTypeStr=single
  Sum : Sum  Inputs=|++  OutDataTypeStr=single
  Sum1 : Sum  Inputs=|-+  OutDataTypeStr=single
  D : Outport  OutDataTypeStr=single
  Q : Outport  Port=2  OutDataTypeStr=single
  wires:
  Beta/1 -> Product3/1, Product1/1
  Alpha/1 -> Product2/1, Product/1
  Theta/1 -> Sin1/1, Sin/1
  Sin1/1 -> Product/2, Product3/2
  Sin/1 -> Product1/2, Product2/2
  Product/1 -> Sum/1
  Product1/1 -> Sum/2
  Sum/1 -> D/1
  Product2/1 -> Sum1/1
  Product3/1 -> Sum1/2
  Sum1/1 -> Q/1

== system FocESMOGenerator/FocSensorLess_ASMO/SVPWM ==
  Ualpha : Inport  OutDataTypeStr=single
  Ubeta : Inport  Port=2  OutDataTypeStr=single
  UBus : Inport  Port=3  OutDataTypeStr=single
  Constant : Constant  Value=0.5  OutDataTypeStr=single
  Divide : Product  Inputs=*/  OutDataTypeStr=single
  Gain : Gain  Gain=-1  OutDataTypeStr=single
  InvClark : Subsystem
  Mux : Mux  Inputs=3
  Sum : Sum  Inputs=++|  OutDataTypeStr=single
  Sum1 : Sum  Inputs=|++  OutDataTypeStr=single
  ei_t : Subsystem
  Tabc : Outport  OutDataTypeStr=single
  wires:
  Ualpha/1 -> InvClark/1(Ualpha)
  Ubeta/1 -> InvClark/2(Ubeta)
  ei_t/1(ei_t) -> Sum/1
  InvClark/1(Ua) -> Mux/1
  InvClark/2(Ub) -> Mux/2
  InvClark/3(Uc) -> Mux/3
  Sum/1 -> Gain/1
  Mux/1 -> Sum/2, ei_t/1(Uabc)
  Divide/1 -> Sum1/1
  Constant/1 -> Sum1/2
  UBus/1 -> Divide/2
  Gain/1 -> Divide/1
  Sum1/1 -> Tabc/1

== system FocESMOGenerator/FocSensorLess_ASMO/Subsystem1 ==
  Id_Ref : Inport
  Id_Real : Inport  Port=2
  Iq_Real : Inport  Port=3
  Iq_Ref : Inport  Port=4
  Current_Kp : Inport  Port=5
  Current_Ki : Inport  Port=6
  Discrete PID Controller : slpidlib/PID Controller  Controller=PI  Form=Parallel  TimeDomain=Discrete-time  UseExternalTs=off  SampleTime=-1  IntegratorMethod=Forward Euler  FilterMethod=Forward Euler  ControllerParametersSource=external  P=1  I=1  UseKiTs=off  D=0  UseExternalDerivativeSource=off  N=100  UseFilter=on  TunerSelectOption=Transfer Function Based (PID Tuner App)  InitialConditionSource=internal  InitialConditionForIntegrator=0  InitialConditionForFilter=0  DifferentiatorICPrevScaledInput=0  ExternalReset=none  TrackingMode=off  Kt=1  LimitOutput=on  SatLimitsSource=internal  UpperSaturationLimit=6  LowerSaturationLimit=-6  LinearizeAsGain=off  AntiWindupMode=clamping  Kb=1  LimitIntegrator=off  UpperIntegratorSaturationLimit=inf  LowerIntegratorSaturationLimit=-inf  SaturateOnIntegerOverflow=on  PGainOutDataTypeStr=single  PProdOutDataTypeStr=single  POutMin=[]  POutMax=[]  IGainOutDataTypeStr=single  IProdOutDataTypeStr=single  IOutMin=[]  IOutMax=[]  DOutMin=[]  DOutMax=[]  NOutMin=[]  NOutMax=[]  SumOutDataTypeStr=single  SumOutMin=[]  SumOutMax=[]  SaturationOutMin=[]  SaturationOutMax=[]  PParamMin=[]  PParamMax=[]  IParamMin=[]  IParamMax=[]  DParamMin=[]  DParamMax=[]  NParamMin=[]  NParamMax=[]  KbParamMin=[]  KbParamMax=[]  KtParamMin=[]  KtParamMax=[]  KbOutMin=[]  KbOutMax=[]  KtOutMin=[]  KtOutMax=[]  IntegratorOutMin=[]  IntegratorOutMax=[]  FilterOutMin=[]  FilterOutMax=[]  SumI1OutMin=[]  SumI1OutMax=[]  SumI2OutMin=[]  SumI2OutMax=[]  SumI3OutMin=[]  SumI3OutMax=[]  SumI4OutMin=[]  SumI4OutMax=[]  SumDOutMin=[]  SumDOutMax=[]  DifferentiatorOutMin=[]  DifferentiatorOutMax=[]  FilterDiffOutCoefMin=[]  FilterDiffOutCoefMax=[]  ReciprocalOutMin=[]  ReciprocalOutMax=[]  SumDenOutMin=[]  SumDenOutMax=[]  SumNumOutMin=[]  SumNumOutMax=[]  DivideOutMin=[]  DivideOutMax=[]  UdiffTsProdOutMin=[]  UdiffTsProdOutMax=[]  NTsProdOutMin=[]  NTsProdOutMax=[]  UintegralTsProdOutMin=[]  UintegralTsProdOutMax=[]  UngainTsProdOutMin=[]  UngainTsProdOutMax=[]  ClampingZeroOutDataTypeStr=Inherit: Inherit via back propagation  ClampingZeroOutMin=[]  ClampingZeroOutMax=[]  FilterDenConstantOutDataTypeStr=Inherit: Inherit via back propagation  FilterDenConstantOutMin=[]  FilterDenConstantOutMax=[]  PCopyOutDataTypeStr=Inherit: Inherit via back propagation  PCopyOutMin=[]  PCopyOutMax=[]  NCopyOutDataTypeStr=Inherit: Inherit via back propagation  NCopyOutMin=[]  NCopyOutMax=[]  IntegratorContinuousStateAttributes=''  IntegratorStateMustResolveToSignalObject=off  IntegratorRTWStateStorageClass=Auto  FilterContinuousStateAttributes=''  FilterStateMustResolveToSignalObject=off  FilterRTWStateStorageClass=Auto  ParallelPVariant=ExternalParameters  IdealPVariant=Disabled  IVariant=ExternalParameters  DVariant=Disabled  IntegratorVariant=Discrete  SatVariant=Enabled  AWVariant=DiscClampingParallel  PCopyVariant=Disabled  TRVariant=Disabled  FdbkBlocksVariant=Forward  IdealPFdbkVariant=Disabled  SatFdbkVariant=Disabled  DerivativeFilterVariant=Disabled  NVariant=Disabled  NCopyVariant=Disabled_SignalSpec  FilterICVariant=Disabled  IntegratorICVariant=InternalICs  ExternalResetVariant=Disabled  TRSumVariant=Passthrough  SumFdbkVariant=Disabled  SumVariant=Sum_PI  TsampFilterVariant=InternalTs  TsampNgainVariant=Passthrough  TsampIntegralVariant=Disabled_SignalSpec  ExternalSaturationOutDataTypeStr=Inherit: Same as second input  DerivativeSourceVariant=Disabled
      settings: LibrarySourceBlock=simulink/Discrete/Discrete PID Controller
  Discrete PID Controller1 : slpidlib/PID Controller  Controller=PI  Form=Parallel  TimeDomain=Discrete-time  UseExternalTs=off  SampleTime=-1  IntegratorMethod=Forward Euler  FilterMethod=Forward Euler  ControllerParametersSource=external  P=1  I=1  UseKiTs=off  D=0  UseExternalDerivativeSource=off  N=100  UseFilter=on  TunerSelectOption=Transfer Function Based (PID Tuner App)  InitialConditionSource=internal  InitialConditionForIntegrator=0  InitialConditionForFilter=0  DifferentiatorICPrevScaledInput=0  ExternalReset=none  TrackingMode=off  Kt=1  LimitOutput=on  SatLimitsSource=internal  UpperSaturationLimit=6  LowerSaturationLimit=-6  LinearizeAsGain=off  AntiWindupMode=clamping  Kb=1  LimitIntegrator=off  UpperIntegratorSaturationLimit=inf  LowerIntegratorSaturationLimit=-inf  SaturateOnIntegerOverflow=on  PGainOutDataTypeStr=single  PProdOutDataTypeStr=single  POutMin=[]  POutMax=[]  IGainOutDataTypeStr=single  IProdOutDataTypeStr=single  IOutMin=[]  IOutMax=[]  DOutMin=[]  DOutMax=[]  NOutMin=[]  NOutMax=[]  SumOutDataTypeStr=single  SumOutMin=[]  SumOutMax=[]  SaturationOutMin=[]  SaturationOutMax=[]  PParamMin=[]  PParamMax=[]  IParamMin=[]  IParamMax=[]  DParamMin=[]  DParamMax=[]  NParamMin=[]  NParamMax=[]  KbParamMin=[]  KbParamMax=[]  KtParamMin=[]  KtParamMax=[]  KbOutMin=[]  KbOutMax=[]  KtOutMin=[]  KtOutMax=[]  IntegratorOutMin=[]  IntegratorOutMax=[]  FilterOutMin=[]  FilterOutMax=[]  SumI1OutMin=[]  SumI1OutMax=[]  SumI2OutMin=[]  SumI2OutMax=[]  SumI3OutMin=[]  SumI3OutMax=[]  SumI4OutMin=[]  SumI4OutMax=[]  SumDOutMin=[]  SumDOutMax=[]  DifferentiatorOutMin=[]  DifferentiatorOutMax=[]  FilterDiffOutCoefMin=[]  FilterDiffOutCoefMax=[]  ReciprocalOutMin=[]  ReciprocalOutMax=[]  SumDenOutMin=[]  SumDenOutMax=[]  SumNumOutMin=[]  SumNumOutMax=[]  DivideOutMin=[]  DivideOutMax=[]  UdiffTsProdOutMin=[]  UdiffTsProdOutMax=[]  NTsProdOutMin=[]  NTsProdOutMax=[]  UintegralTsProdOutMin=[]  UintegralTsProdOutMax=[]  UngainTsProdOutMin=[]  UngainTsProdOutMax=[]  ClampingZeroOutDataTypeStr=Inherit: Inherit via back propagation  ClampingZeroOutMin=[]  ClampingZeroOutMax=[]  FilterDenConstantOutDataTypeStr=Inherit: Inherit via back propagation  FilterDenConstantOutMin=[]  FilterDenConstantOutMax=[]  PCopyOutDataTypeStr=Inherit: Inherit via back propagation  PCopyOutMin=[]  PCopyOutMax=[]  NCopyOutDataTypeStr=Inherit: Inherit via back propagation  NCopyOutMin=[]  NCopyOutMax=[]  IntegratorContinuousStateAttributes=''  IntegratorStateMustResolveToSignalObject=off  IntegratorRTWStateStorageClass=Auto  FilterContinuousStateAttributes=''  FilterStateMustResolveToSignalObject=off  FilterRTWStateStorageClass=Auto  ParallelPVariant=ExternalParameters  IdealPVariant=Disabled  IVariant=ExternalParameters  DVariant=Disabled  IntegratorVariant=Discrete  SatVariant=Enabled  AWVariant=DiscClampingParallel  PCopyVariant=Disabled  TRVariant=Disabled  FdbkBlocksVariant=Forward  IdealPFdbkVariant=Disabled  SatFdbkVariant=Disabled  DerivativeFilterVariant=Disabled  NVariant=Disabled  NCopyVariant=Disabled_SignalSpec  FilterICVariant=Disabled  IntegratorICVariant=InternalICs  ExternalResetVariant=Disabled  TRSumVariant=Passthrough  SumFdbkVariant=Disabled  SumVariant=Sum_PI  TsampFilterVariant=InternalTs  TsampNgainVariant=Passthrough  TsampIntegralVariant=Disabled_SignalSpec  ExternalSaturationOutDataTypeStr=Inherit: Same as second input  DerivativeSourceVariant=Disabled
      settings: LibrarySourceBlock=simulink/Discrete/Discrete PID Controller
  Sum : Sum  Inputs=+-|
  Sum1 : Sum  Inputs=+-|
  IqPID_Out : Outport
  IdPID_Out : Outport  Port=2
  wires:
  Sum/1 -> Discrete PID Controller/1
  Current_Kp/1 -> Discrete PID Controller/2, Discrete PID Controller1/2
  Iq_Ref/1 -> Sum/1
  Discrete PID Controller/1 -> IqPID_Out/1
  Current_Ki/1 -> Discrete PID Controller/3, Discrete PID Controller1/3
  Iq_Real/1 -> Sum/2
  Id_Ref/1 -> Sum1/1
  Id_Real/1 -> Sum1/2
  Sum1/1 -> Discrete PID Controller1/1
  Discrete PID Controller1/1 -> IdPID_Out/1

== system FocESMOGenerator/FocSensorLess_ASMO/Subsystem2 ==
  Speed_Real : Inport
  Speed_Ref : Inport  Port=2
  Speed_Kp : Inport  Port=3
  Speed_Ki : Inport  Port=4
  Discrete PID Controller : slpidlib/PID Controller  Controller=PI  Form=Parallel  TimeDomain=Discrete-time  UseExternalTs=off  SampleTime=0.00025  IntegratorMethod=Forward Euler  FilterMethod=Forward Euler  ControllerParametersSource=external  P=1  I=1  UseKiTs=off  D=0  UseExternalDerivativeSource=off  N=100  UseFilter=on  TunerSelectOption=Transfer Function Based (PID Tuner App)  InitialConditionSource=internal  InitialConditionForIntegrator=0  InitialConditionForFilter=0  DifferentiatorICPrevScaledInput=0  ExternalReset=none  TrackingMode=off  Kt=1  LimitOutput=on  SatLimitsSource=internal  UpperSaturationLimit=Max_Current  LowerSaturationLimit=-Max_Current  LinearizeAsGain=off  AntiWindupMode=clamping  Kb=1  LimitIntegrator=off  UpperIntegratorSaturationLimit=inf  LowerIntegratorSaturationLimit=-inf  SaturateOnIntegerOverflow=on  PGainOutDataTypeStr=single  PProdOutDataTypeStr=single  POutMin=[]  POutMax=[]  IGainOutDataTypeStr=single  IProdOutDataTypeStr=single  IOutMin=[]  IOutMax=[]  DOutMin=[]  DOutMax=[]  NOutMin=[]  NOutMax=[]  SumOutDataTypeStr=single  SumOutMin=[]  SumOutMax=[]  SaturationOutMin=[]  SaturationOutMax=[]  PParamMin=[]  PParamMax=[]  IParamMin=[]  IParamMax=[]  DParamMin=[]  DParamMax=[]  NParamMin=[]  NParamMax=[]  KbParamMin=[]  KbParamMax=[]  KtParamMin=[]  KtParamMax=[]  KbOutMin=[]  KbOutMax=[]  KtOutMin=[]  KtOutMax=[]  IntegratorOutMin=[]  IntegratorOutMax=[]  FilterOutMin=[]  FilterOutMax=[]  SumI1OutMin=[]  SumI1OutMax=[]  SumI2OutMin=[]  SumI2OutMax=[]  SumI3OutMin=[]  SumI3OutMax=[]  SumI4OutMin=[]  SumI4OutMax=[]  SumDOutMin=[]  SumDOutMax=[]  DifferentiatorOutMin=[]  DifferentiatorOutMax=[]  FilterDiffOutCoefMin=[]  FilterDiffOutCoefMax=[]  ReciprocalOutMin=[]  ReciprocalOutMax=[]  SumDenOutMin=[]  SumDenOutMax=[]  SumNumOutMin=[]  SumNumOutMax=[]  DivideOutMin=[]  DivideOutMax=[]  UdiffTsProdOutMin=[]  UdiffTsProdOutMax=[]  NTsProdOutMin=[]  NTsProdOutMax=[]  UintegralTsProdOutMin=[]  UintegralTsProdOutMax=[]  UngainTsProdOutMin=[]  UngainTsProdOutMax=[]  ClampingZeroOutDataTypeStr=Inherit: Inherit via back propagation  ClampingZeroOutMin=[]  ClampingZeroOutMax=[]  FilterDenConstantOutDataTypeStr=Inherit: Inherit via back propagation  FilterDenConstantOutMin=[]  FilterDenConstantOutMax=[]  PCopyOutDataTypeStr=Inherit: Inherit via back propagation  PCopyOutMin=[]  PCopyOutMax=[]  NCopyOutDataTypeStr=Inherit: Inherit via back propagation  NCopyOutMin=[]  NCopyOutMax=[]  IntegratorContinuousStateAttributes=''  IntegratorStateMustResolveToSignalObject=off  IntegratorRTWStateStorageClass=Auto  FilterContinuousStateAttributes=''  FilterStateMustResolveToSignalObject=off  FilterRTWStateStorageClass=Auto  ParallelPVariant=ExternalParameters  IdealPVariant=Disabled  IVariant=ExternalParameters  DVariant=Disabled  IntegratorVariant=Discrete  SatVariant=Enabled  AWVariant=DiscClampingParallel  PCopyVariant=Disabled  TRVariant=Disabled  FdbkBlocksVariant=Forward  IdealPFdbkVariant=Disabled  SatFdbkVariant=Disabled  DerivativeFilterVariant=Disabled  NVariant=Disabled  NCopyVariant=Disabled_SignalSpec  FilterICVariant=Disabled  IntegratorICVariant=InternalICs  ExternalResetVariant=Disabled  TRSumVariant=Passthrough  SumFdbkVariant=Disabled  SumVariant=Sum_PI  TsampFilterVariant=InternalTs  TsampNgainVariant=Passthrough  TsampIntegralVariant=Disabled_SignalSpec  ExternalSaturationOutDataTypeStr=Inherit: Same as second input  DerivativeSourceVariant=Disabled
      settings: LibrarySourceBlock=simulink/Discrete/Discrete PID Controller
  Sum : Sum  Inputs=+-|
  SpeedPID_Out : Outport
  wires:
  Sum/1 -> Discrete PID Controller/1
  Speed_Kp/1 -> Discrete PID Controller/2
  Speed_Ref/1 -> Sum/1
  Discrete PID Controller/1 -> SpeedPID_Out/1
  Speed_Ki/1 -> Discrete PID Controller/3
  Speed_Real/1 -> Sum/2

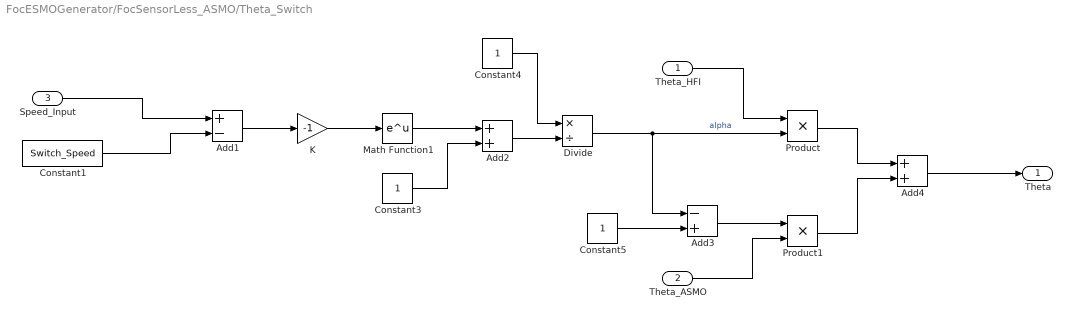
== system FocESMOGenerator/FocSensorLess_ASMO/Theta_Switch ==
  Theta_HFI : Inport
  Theta_ASMO : Inport  Port=2
  Speed_Input : Inport  Port=3
  Add1 : Sum  Inputs=+-  OutDataTypeStr=single  AccumDataTypeStr=single
  Add2 : Sum
  Add3 : Sum  Inputs=-+  OutDataTypeStr=single  AccumDataTypeStr=single
  Add4 : Sum  OutDataTypeStr=single  AccumDataTypeStr=single
  Constant1 : Constant  Value=Switch_Speed  OutDataTypeStr=single
  Constant3 : Constant  OutDataTypeStr=single
  Constant4 : Constant  OutDataTypeStr=single
  Constant5 : Constant  OutDataTypeStr=single
  Divide : Product  Inputs=*/  OutDataTypeStr=single
  K : Gain  Gain=-1  OutDataTypeStr=single
  Math Function1 : Math
  Product : Product  OutDataTypeStr=single
  Product1 : Product  OutDataTypeStr=single
  Theta : Outport
  wires:
  Divide/1 -> Product/2, Add3/1  "alpha"
  Add3/1 -> Product1/1
  Math Function1/1 -> Add2/1
  Add1/1 -> K/1
  Theta_HFI/1 -> Product/1
  Add4/1 -> Theta/1
  Theta_ASMO/1 -> Product1/2
  Constant1/1 -> Add1/2
  Product/1 -> Add4/1
  Constant4/1 -> Divide/1
  Product1/1 -> Add4/2
  Speed_Input/1 -> Add1/1
  Add2/1 -> Divide/2
  Constant3/1 -> Add2/2
  K/1 -> Math Function1/1
  Constant5/1 -> Add3/2

== system FocESMOGenerator/FocSensorLess_ASMO/ASMO/Sigmoid ==
  In1 : Inport
  Add : Sum  OutDataTypeStr=single  AccumDataTypeStr=single
  Add1 : Sum  Inputs=+-  OutDataTypeStr=single  AccumDataTypeStr=single
  Constant : Constant  OutDataTypeStr=single
  Constant1 : Constant  Value=2  OutDataTypeStr=single
  Constant2 : Constant  OutDataTypeStr=single
  Divide : Product  Inputs=*/  OutDataTypeStr=single
  Gain : Gain  Gain=-1  OutDataTypeStr=single
  Math Function : Math
  Out1 : Outport
  wires:
  In1/1 -> Gain/1
  Gain/1 -> Math Function/1
  Math Function/1 -> Add/1
  Constant/1 -> Add/2
  Add/1 -> Divide/2
  Constant1/1 -> Divide/1
  Divide/1 -> Add1/1
  Constant2/1 -> Add1/2
  Add1/1 -> Out1/1

== system FocESMOGenerator/FocSensorLess_ASMO/ASMO/Sigmoid1 ==
  In1 : Inport
  Add : Sum  OutDataTypeStr=single  AccumDataTypeStr=single
  Add1 : Sum  Inputs=+-  OutDataTypeStr=single  AccumDataTypeStr=single
  Constant : Constant  OutDataTypeStr=single
  Constant1 : Constant  Value=2  OutDataTypeStr=single
  Constant2 : Constant  OutDataTypeStr=single
  Divide : Product  Inputs=*/  OutDataTypeStr=single
  Gain : Gain  Gain=-1  OutDataTypeStr=single
  Math Function : Math
  Out1 : Outport
  wires:
  In1/1 -> Gain/1
  Gain/1 -> Math Function/1
  Math Function/1 -> Add/1
  Constant/1 -> Add/2
  Add/1 -> Divide/2
  Constant1/1 -> Divide/1
  Divide/1 -> Add1/1
  Constant2/1 -> Add1/2
  Add1/1 -> Out1/1

== system FocESMOGenerator/FocSensorLess_ASMO/ASMO_PLL/Subsystem ==
  In1 : Inport
  Add : Sum  OutDataTypeStr=single  AccumDataTypeStr=single
  Constant1 : Constant  Value=pi  OutDataTypeStr=single
  Constant2 : Constant  Value=2*pi  OutDataTypeStr=single
  Mod1 : Math  Operator=mod
  Out1 : Outport
  wires:
  Constant1/1 -> Add/2
  Add/1 -> Mod1/1
  Mod1/1 -> Out1/1
  Constant2/1 -> Mod1/2
  In1/1 -> Add/1

== system FocESMOGenerator/FocSensorLess_ASMO/HFI_Inject/Subsystem ==
  Add : Sum
  Constant1 : Constant  Value=-UdInjectVal  OutDataTypeStr=single
  Constant2 : Constant  Value=0  OutDataTypeStr=single
  Constant6 : Constant  Value=UdInjectVal  OutDataTypeStr=single
  If : If  IfExpression=u1 == 1  ElseIfExpressions=u1 == 0
  If Action Subsystem : Subsystem  TreatAsAtomicUnit=on
  If Action Subsystem1 : Subsystem  TreatAsAtomicUnit=on
  If Action Subsystem2 : Subsystem  TreatAsAtomicUnit=on
  Merge : Merge  Inputs=3
  Pulse Generator : DiscretePulseGenerator  PulseType=Time based  Period=0.0001  PulseWidth=50  PhaseDelay=0.2
  Scope : Scope
  Step : Step  Time=0.2  Before=5  After=0  SampleTime=0
  Ud_Inject : Outport
  wires:
  Merge/1 -> Ud_Inject/1
  Constant1/1 -> If Action Subsystem1/1(In1)
  If Action Subsystem/1(Output) -> Merge/1
  If Action Subsystem1/1(Output) -> Merge/2
  Constant6/1 -> If Action Subsystem/1(In1)
  Pulse Generator/1 -> Add/1
  Add/1 -> Scope/1, If/1
  Step/1 -> Add/2
  If/1 -> If Action Subsystem/Action
  If/2 -> If Action Subsystem1/Action
  If/3 -> If Action Subsystem2/Action
  If Action Subsystem2/1(Output) -> Merge/3
  Constant2/1 -> If Action Subsystem2/1(In1)

== system FocESMOGenerator/FocSensorLess_ASMO/HFI_Inject/Subsystem4 ==
  Add1 : Sum  Inputs=+-  OutDataTypeStr=single  AccumDataTypeStr=single
  Add2 : Sum  Inputs=+-  OutDataTypeStr=single  AccumDataTypeStr=single
  Scope : Scope
  Scope1 : Scope
  Scope2 : Scope
  Step1 : Step  Time=0.13  After=-2  OutDataTypeStr=single  SampleTime=0
  Step2 : Step  Time=0.14  After=-2  OutDataTypeStr=single  SampleTime=0
  Step3 : Step  Time=0.1  After=2  OutDataTypeStr=single  SampleTime=0
  Step4 : Step  Time=0.11  After=2  OutDataTypeStr=single  SampleTime=0
  Sum : Sum  Inputs=+|+
  NDS_Signal : Outport
  wires:
  Add2/1 -> Sum/2, Scope1/1
  Step1/1 -> Add2/1
  Step2/1 -> Add2/2
  Step3/1 -> Add1/1
  Add1/1 -> Sum/1, Scope/1
  Step4/1 -> Add1/2
  Sum/1 -> Scope2/1, NDS_Signal/1

== system FocESMOGenerator/FocSensorLess_ASMO/NSD/Subsystem ==
  Input : Inport
  Trigger : TriggerPort  VariantControl=(inherit)  PortDimensions=1
  Output : Outport
  wires:
  Input/1 -> Output/1
